simulink model "state_space_simulink"  (R2019a)
settings: Solver=VariableStepAuto  StartTime=0.0  StopTime=2  RelTol=1e-3
values from neighbouring files (symbols this model uses):
  A = [ 0   1   0 ... (first row only)    [state_space_controller.m]
  B = [ 0 ... (first row only)    [state_space_controller.m]
  K = place(A,B,[p1 p2 p3])    [state_space_controller.m]
  Nbar = rscale(A, B, C, 0, K)    [state_space_controller.m]
settings Model: Creator=USER  LastModifiedBy=USER

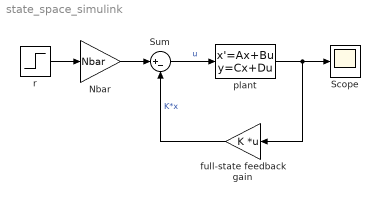
== system state_space_simulink ==
  Nbar : Gain  Gain=Nbar
  Scope : Scope
  Sum : Sum  Inputs=|+-
  full-state feedback gain : Gain  Gain=K  Multiplication=Matrix(K*u)
  plant : StateSpace  A=A  B=B  C=eye(3)  D=[0;0;0]  InitialCondition=0
  r : Step  Time=0  After=0.001  SampleTime=0
  wires:
  plant/1 -> full-state feedback gain/1, Scope/1
  Sum/1 -> plant/1  "u"
  full-state feedback gain/1 -> Sum/2  "K*x"
  r/1 -> Nbar/1
  Nbar/1 -> Sum/1
